simulink model "ThereBoard"  (R2019b)
settings: Solver=FixedStepAuto  StartTime=0.0  StopTime=10.0  RelTol=1e-3
undefined symbols (not defined in the file): A9, BF, CB
libraries: androiduilib x7, androidcommunicationlib x1, androidaudiovideolib x1, androidsensorlib x1
settings Model: Creator=The MathWorks, Inc.  LastModifiedBy=matte
settings DataIOCC: ReturnWorkspaceOutputs=off
settings OptimizationCC: PassReuseOutputArgsThreshold=0  MaxStackSize=64
settings DebuggingCC: ParameterTunabilityLossMsg=error  ArithmeticOperatorsInVariantConditions=warning
settings HardwareCC: ProdBitPerPointer=32  ProdBitPerSizeT=32  ProdBitPerPtrDiffT=32  ProdLargestAtomicInteger=Long  ProdLargestAtomicFloat=Double  ProdWordSize=32  ProdHWDeviceType=ARM Compatible->ARM Cortex  UseEmbeddedCoderFeatures=off  UseSimulinkCoderFeatures=off
settings SFSimCC: SimUseLocalCustomCode=off  MATLABDynamicMemAlloc=off  CustomCodeUndefinedFunction=UseInterfaceOnly
settings RTWCC: SystemTargetFile=ert.tlc  HardwareBoard=Android Device  TLCOptions="-aInlineSetEventsForThisBaseRateFcn=TLC_FALSE -aSuppressMultiTaskScheduler=TLC_FALSE  -aRateBasedStepFcn=0"  TemplateMakefile=ert_default_tmf  GenerateReport=on  RTWUseLocalCustomCode=off  Toolchain=Android SDK/NDK Tools  LaunchReport=on
settings CodeAppCC: ForceParamTrailComments=on  OperatorAnnotations=on
settings ERTTargetCC: ERTCustomFileBanners=off  SupportContinuousTime=on  SupportNonInlinedSFcns=on  RemoveResetFunc=off  ModelStepFunctionPrototypeControlCompliant=off

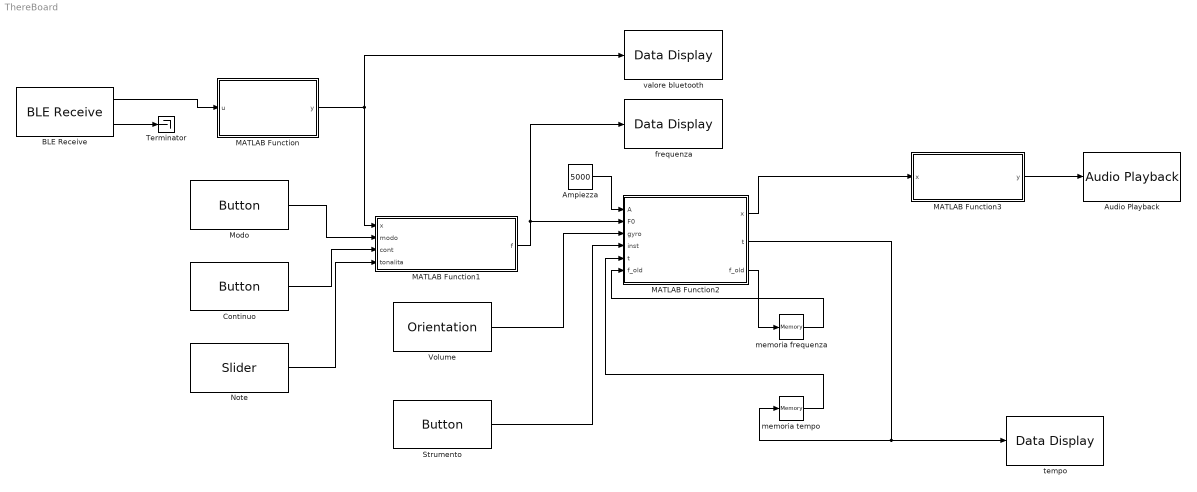
== system ThereBoard ==
  " BLE Receive" : androidcommunicationlib/BLE Receive  DeviceMode=Central (Client)  BluetoothAddress=CB:60:BF:A9:53:3E  CharUUID=00002a37-0000-1000-8000-00805f9b34fb  ServiceUUID=0000180d-0000-1000-8000-00805f9b34fb  device=ThereBoard  character="Heart Rate\\Heart Rate  Measurement"  CustomService=off  ServiceName=Heart Rate  CharacteristicName="Heart Rate  Measurement"  CustomServiceUUID=<Enter Service UUID>  CustomCharUUID=<Enter Characteristic UUID>  DataSize=3  SampleTime=0.001  charseruuid=00001801-0000-1000-8000-00805f9b34fb\00002a05-0000-1000-8000-00805f9b34fb  seruuid=00001810-0000-1000-8000-00805f9b34fb  PeripheralService=0000180d-0000-1000-8000-00805f9b34fb  PeripheralCharacteristic=00002a37-0000-1000-8000-00805f9b34fb  chruuid=00002a37-0000-1000-8000-00805f9b34fb  BLEId=ThereBoard/_BLE_Receive  Devicename=ThereBoard  IsCustomService=0
      settings: SourceProductName=Simulink Support Package for Android Devices  SourceProductBaseCode=ANDROID
  Ampiezza : Constant  Value=5000  OutDataTypeStr=int32
  Audio Playback : androidaudiovideolib/Audio Playback  SampleFreq=8000  AudioSamplingFreq=8000  SampleTime=0.1  DeviceStr=0  QueueDuration=0  BlockPlatform=Android
      settings: SourceProductName=Simulink Support Package for Android Devices  SourceProductBaseCode=ANDROID
  Continuo : androiduilib/Button  ButtonState=Not pressed  ButtonId=ThereBoard/Continuo  State=off  SampleTime=0.1  BlockPlatform=Android
      settings: SourceProductName=Simulink Support Package for Android Devices  SourceProductBaseCode=ANDROID
  MATLAB Function : MATLAB Function  TreatAsAtomicUnit=on
  MATLAB Function1 : MATLAB Function  TreatAsAtomicUnit=on
  MATLAB Function2 : MATLAB Function  TreatAsAtomicUnit=on
  MATLAB Function3 : MATLAB Function  TreatAsAtomicUnit=on
  Modo : androiduilib/Button  ButtonState=Not pressed  ButtonId=ThereBoard/Modo  State=off  SampleTime=0.1  BlockPlatform=Android
      settings: SourceProductName=Simulink Support Package for Android Devices  SourceProductBaseCode=ANDROID
  Note : androiduilib/Slider  Min=1  Value=1  Max=12  Resolution=1  SliderId=ThereBoard/Note  SampleTime=0.1  BlockPlatform=Android
      settings: SourceProductName=Simulink Support Package for Android Devices  SourceProductBaseCode=ANDROID
  Strumento : androiduilib/Button  ButtonState=Not pressed  ButtonId=ThereBoard/Strumento  State=off  SampleTime=0.1  BlockPlatform=Android
      settings: SourceProductName=Simulink Support Package for Android Devices  SourceProductBaseCode=ANDROID
  Terminator : Terminator
  Volume : androidsensorlib/Orientation  SampleTime=0.1  SimulateUsing=Code generation
      settings: SourceProductName=Simulink Support Package for Android Devices  SourceProductBaseCode=ANDROID
  frequenza : androiduilib/Data Display  DataDisplayId=ThereBoard/frequenza  Format=Float  Precision=6  SimulateUsing=Code generation  blockPlatform=Android
      settings: SourceProductName=Simulink Support Package for Android Devices  SourceProductBaseCode=ANDROID
  memoria frequenza : Memory  InheritSampleTime=on  LinearizeMemory=on  LinearizeAsDelay=on
  memoria tempo : Memory  InheritSampleTime=on  LinearizeMemory=on  LinearizeAsDelay=on
  tempo : androiduilib/Data Display  DataDisplayId=ThereBoard/tempo  Format=Float  Precision=3  SimulateUsing=Code generation  blockPlatform=Android
      settings: SourceProductName=Simulink Support Package for Android Devices  SourceProductBaseCode=ANDROID
  valore bluetooth : androiduilib/Data Display  DataDisplayId=ThereBoard/valore_bluetooth  Format=Integer  Precision=6  SimulateUsing=Code generation  blockPlatform=Android
      settings: SourceProductName=Simulink Support Package for Android Devices  SourceProductBaseCode=ANDROID
  wires:
  " BLE Receive"/1 -> MATLAB Function/1(u)
  " BLE Receive"/2 -> Terminator/1
  MATLAB Function/1(y) -> MATLAB Function1/1(x), valore bluetooth/1
  MATLAB Function2/2(t) -> memoria tempo/1, tempo/1
  memoria tempo/1 -> MATLAB Function2/5("t ")
  MATLAB Function2/3(f_old) -> memoria frequenza/1
  memoria frequenza/1 -> MATLAB Function2/6("f_old ")
  MATLAB Function2/1(x) -> MATLAB Function3/1(x)
  Ampiezza/1 -> MATLAB Function2/1(A)
  MATLAB Function1/1(f) -> MATLAB Function2/2(F0), frequenza/1
  MATLAB Function3/1(y) -> Audio Playback/1
  Modo/1 -> MATLAB Function1/2(modo)
  Note/1 -> MATLAB Function1/4(tonalita)
  Volume/1 -> MATLAB Function2/3(gyro)
  Strumento/1 -> MATLAB Function2/4(inst)
  Continuo/1 -> MATLAB Function1/3(cont)

== matlab function ThereBoard/MATLAB Function ==
  data: u input; y output
function y  = concat_bytes(u)

    x1 = toUintVal(u(2));
    x2 = toUintVal(u(3));

    y  = x1 + bitsll(x2, 8);

end

function uintval = toUintVal(val)
%{
dato un intero su 8 bit, 
- se positivo lo restituisce come int16
- se negativo lo interpreta come intero positivo.

esempio:
84  = 0101 0100 bin -> 84
-84 = 1010 1100 bin -> 172

%}
    uintval = int32(bitand(val, int8(127)));
    if val < 0
        uintval = bitor(uintval, int32(128));
    end

end

== matlab function ThereBoard/MATLAB Function1 ==
  data: x input; f output; modo input; cont input; tonalita input
function f = dist_to_frequency(x, modo, cont, tonalita)

if cont == 0
    note = 0;
    switch tonalita
        case 1
            note = 261.63;
        case 2
            note = 277.18;
        case 3
            note = 293.66;
        case 4
            note = 311.13;
        case 5
            note = 329.63;
        case 6
            note = 349.23;
        case 7
            note = 369.99;
        case 8
            note = 392;
        case 9
            note = 415.30;
        case 10
            note = 440;
        case 11
            note = 466.16;
        case 12
            note = 493.88;
    end

    if modo == 0

        if x<=10
            f = double(90);
        elseif x>10 && x<60
            f = double(note/2^(1/12));
        elseif x>=60 && x<100
            f = double(note);
        elseif x>=100 && x<140
            f = double(note*2^(2/12));
        elseif x>=140 && x<180
            f = double(note*2^(4/12));
        elseif x>=180 && x<220
            f = double(note*2^(5/12));
        elseif x>=220 && x<260
            f = double(note*2^(7/12));
        elseif x>=260 && x<300
            f = double(note*2^(9/12));
        elseif x>=300 && x<340
            f = double(note*2^(11/12));
        else
            f = double(note*2);

        end
    else
        if x<=10
            f = double(90);
        elseif x>10 && x<60
            f = double(note/2^(2/12));
        elseif x>=60 && x<100
            f = double(note);
        elseif x>=100 && x<140
            f = double(note*2^(2/12));
        elseif x>=140 && x<180
            f = double(note*2^(3/12));
        elseif x>=180 && x<220
            f = double(note*2^(5/12));
        elseif x>=220 && x<260
            f = double(note*2^(7/12));
        elseif x>=260 && x<300
            f = double(note*2^(8/12));
        elseif x>=300 && x<340
            f = double(note*2^(10/12));
        else
            f = double(note*2);

        end
    end
else
    if x <= 10 
        f = double(90);
    else
        f = double(233.08+x);
    end
end

== matlab function ThereBoard/MATLAB Function3 ==
  data: x input; y output
function y = mono_to_stereo(x)

y = [x x];

== matlab function ThereBoard/MATLAB Function2 ==
  data: A input; F0 input; gyro input; inst input; x output; t input; t output; f_old input; f_old output
function [x, t, f_old] = sinewave_generator(A, F0, gyro, inst, t, f_old)
%{
Funzione che genera un'onda sinusoidale di
- frequenza F0 [Hz]
- ampiezza A [compresa tra 0 e 32737]

Il risultato è un array di N valori generati partendo dal tempo t calcolato
rispetto alla computazione precedente.
Al termine della computazione il tempo è ridotto di n periodi per limitarne
la crescita.
%}

Fs=8000; %[Hz]
Ts=1/Fs; %[s]
N=8;%[S]
    
x = int16(zeros(N,1));

if F0 > 90
    
    t = f_old * t / F0;
    f_old = F0;
    F1 = 2*F0;
    F2 = 3*F0;
    F3 = 4*F0;
    A1=A/2;
    A2=A/3;
    A3=A/4;

    if gyro(2) > 1
        volinc = double(gyro(2)/10);
    elseif gyro(2) <-1
        volinc = double(-gyro(2)/10);   
    else
        volinc = 1;
    end

    for n=0:N-1
        if inst == 0
            x(n+1)=int16(volinc*(A*sin(2*pi*F0*t*Ts) + A1*sin(2*pi*F1*t*Ts) + A2*sin(2*pi*F2*t*Ts) + A3*sin(2*pi*F3*t*Ts))/4);
        else
            x(n+1)=int16(volinc*A*sin(2*pi*F0*t*Ts));
        end
        t = t + 1;
    end

    T = Fs/F0;
    t = t - T*floor(t/T);
    
else
    t = f_old * t / F0;
    f_old = F0;


    for n=0:N-1
        x(n+1)=0; 
        t = t + 1;
    end

    T = Fs/F0;
    t = t - T*floor(t/T);
end
